simulink model "TST_FlSys_CalcCnvFac"  (R2016b)
settings: Solver=FixedStepDiscrete  StartTime=0.0  StopTime=simTime  FixedStep=sampleTime  RelTol=1e-3
values from neighbouring files (symbols this model uses):
  testCase = 1    [initTST_FlSys_CalcCnvFac_001.m]
libraries: simulink x2
settings Model: Creator=WF305  LastModifiedBy=WF305
settings DebuggingCC: SignalRangeChecking=error

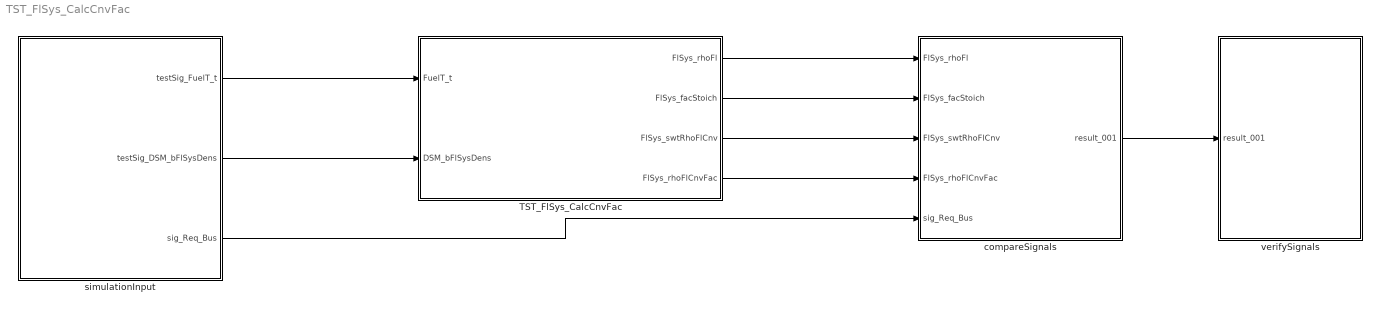
== system TST_FlSys_CalcCnvFac ==
  TST_FlSys_CalcCnvFac : Subsystem
  compareSignals : Subsystem
  simulationInput : Subsystem
  verifySignals : Subsystem
  wires:
  simulationInput/1(testSig_FuelT_t) -> TST_FlSys_CalcCnvFac/1(FuelT_t)
  simulationInput/2(testSig_DSM_bFlSysDens) -> TST_FlSys_CalcCnvFac/2(DSM_bFlSysDens)
  TST_FlSys_CalcCnvFac/1(FlSys_rhoFl) -> compareSignals/1(FlSys_rhoFl)
  TST_FlSys_CalcCnvFac/2(FlSys_facStoich) -> compareSignals/2(FlSys_facStoich)
  TST_FlSys_CalcCnvFac/3(FlSys_swtRhoFlCnv) -> compareSignals/3(FlSys_swtRhoFlCnv)
  TST_FlSys_CalcCnvFac/4(FlSys_rhoFlCnvFac) -> compareSignals/4(FlSys_rhoFlCnvFac)
  simulationInput/3(sig_Req_Bus) -> compareSignals/5(sig_Req_Bus)
  compareSignals/1(result_001) -> verifySignals/1(result_001)

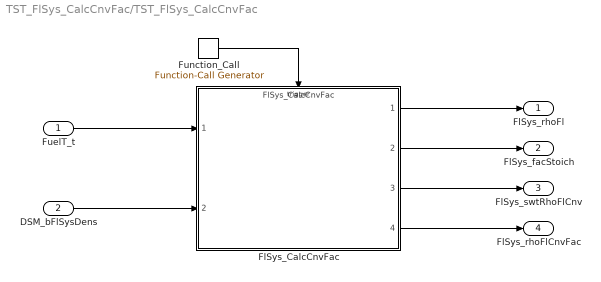
== system TST_FlSys_CalcCnvFac/TST_FlSys_CalcCnvFac ==
  FuelT_t : Inport
  DSM_bFlSysDens : Inport  Port=2
  FlSys_CalcCnvFac : ModelReference  ModelNameDialog=FlSys_CalcCnvFac  ModelReferenceVersion=1.9  TriggerPortName=function  TriggerPortTriggerType=function-call  TriggerPortStatesWhenEnabling=held
  Function_Call : simulink/Ports & Subsystems/Function-Call Generator  sample_time=sampleTime  numberOfIterations=1
  FlSys_rhoFl : Outport
  FlSys_facStoich : Outport  Port=2
  FlSys_swtRhoFlCnv : Outport  Port=3
  FlSys_rhoFlCnvFac : Outport  Port=4
  wires:
  Function_Call/1 -> FlSys_CalcCnvFac/Trigger
  FuelT_t/1 -> FlSys_CalcCnvFac/1
  DSM_bFlSysDens/1 -> FlSys_CalcCnvFac/2
  FlSys_CalcCnvFac/1 -> FlSys_rhoFl/1
  FlSys_CalcCnvFac/2 -> FlSys_facStoich/1
  FlSys_CalcCnvFac/3 -> FlSys_swtRhoFlCnv/1
  FlSys_CalcCnvFac/4 -> FlSys_rhoFlCnvFac/1

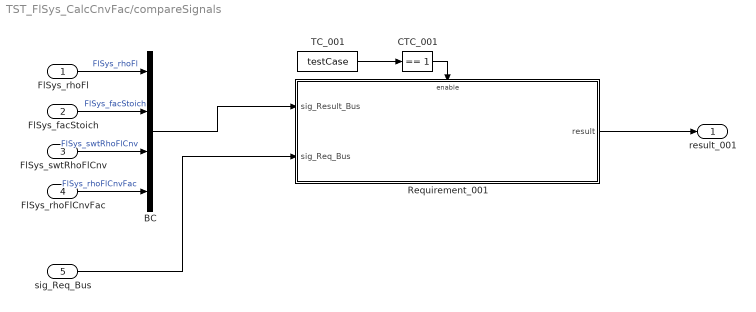
== system TST_FlSys_CalcCnvFac/compareSignals ==
  FlSys_rhoFl : Inport
  FlSys_facStoich : Inport  Port=2
  FlSys_swtRhoFlCnv : Inport  Port=3
  FlSys_rhoFlCnvFac : Inport  Port=4
  sig_Req_Bus : Inport  Port=5
  BC : BusCreator  Inputs=4
  CTC_001 : simulink/Logic and Bit Operations/Compare To Constant  relop===  const=1  OutDataTypeStr=boolean
  Requirement_001 : Subsystem
  TC_001 : Constant  Value=testCase
  result_001 : Outport
  wires:
  FlSys_rhoFl/1 -> BC/1  "FlSys_rhoFl"
  FlSys_facStoich/1 -> BC/2  "FlSys_facStoich"
  FlSys_swtRhoFlCnv/1 -> BC/3  "FlSys_swtRhoFlCnv"
  FlSys_rhoFlCnvFac/1 -> BC/4  "FlSys_rhoFlCnvFac"
  TC_001/1 -> CTC_001/1
  CTC_001/1 -> Requirement_001/Enable
  sig_Req_Bus/1 -> Requirement_001/2(sig_Req_Bus)
  BC/1 -> Requirement_001/1(sig_Result_Bus)
  Requirement_001/1(result) -> result_001/1

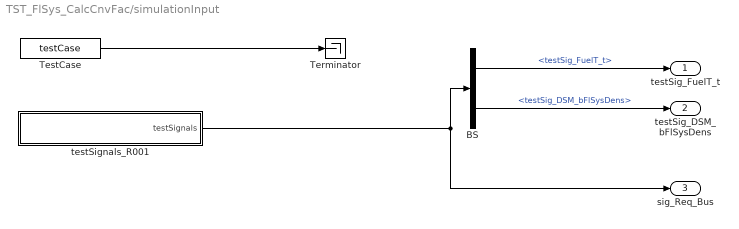
== system TST_FlSys_CalcCnvFac/simulationInput ==
  BS : BusSelector  OutputSignals=testSig_FuelT_t,testSig_DSM_bFlSysDens
  Terminator : Terminator
  TestCase : Constant  Value=testCase
  testSignals_R001 : Subsystem
  testSig_FuelT_t : Outport
  testSig_DSM_bFlSysDens : Outport  Port=2
  sig_Req_Bus : Outport  Port=3
  wires:
  BS/1 -> testSig_FuelT_t/1  "<testSig_FuelT_t>"
  BS/2 -> testSig_DSM_bFlSysDens/1  "<testSig_DSM_bFlSysDens>"
  testSignals_R001/1(testSignals) -> BS/1, sig_Req_Bus/1
  TestCase/1 -> Terminator/1

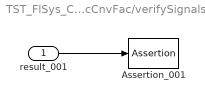
== system TST_FlSys_CalcCnvFac/verifySignals ==
  result_001 : Inport
  Assertion_001 : Assertion
  wires:
  result_001/1 -> Assertion_001/1

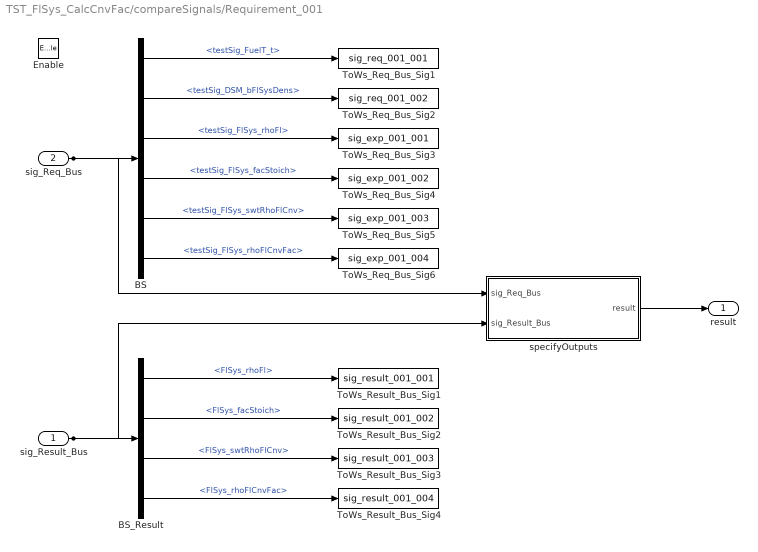
== system TST_FlSys_CalcCnvFac/compareSignals/Requirement_001 ==
  sig_Result_Bus : Inport
  sig_Req_Bus : Inport  Port=2
  Enable : EnablePort
  BS : BusSelector  OutputSignals=testSig_FuelT_t,testSig_DSM_bFlSysDens,testSig_FlSys_rhoFl,testSig_FlSys_facStoich,testSig_FlSys_swtRhoFlCnv,testSig_FlSys_rhoFlCnvFac
  BS_Result : BusSelector  OutputSignals=FlSys_rhoFl,FlSys_facStoich,FlSys_swtRhoFlCnv,FlSys_rhoFlCnvFac
  ToWs_Req_Bus_Sig1 : ToWorkspace  VariableName=sig_req_001_001  SaveFormat=Structure With Time
  ToWs_Req_Bus_Sig2 : ToWorkspace  VariableName=sig_req_001_002  SaveFormat=Structure With Time
  ToWs_Req_Bus_Sig3 : ToWorkspace  VariableName=sig_exp_001_001  SaveFormat=Structure With Time
  ToWs_Req_Bus_Sig4 : ToWorkspace  VariableName=sig_exp_001_002  SaveFormat=Structure With Time
  ToWs_Req_Bus_Sig5 : ToWorkspace  VariableName=sig_exp_001_003  SaveFormat=Structure With Time
  ToWs_Req_Bus_Sig6 : ToWorkspace  VariableName=sig_exp_001_004  SaveFormat=Structure With Time
  ToWs_Result_Bus_Sig1 : ToWorkspace  VariableName=sig_result_001_001  SaveFormat=Structure With Time
  ToWs_Result_Bus_Sig2 : ToWorkspace  VariableName=sig_result_001_002  SaveFormat=Structure With Time
  ToWs_Result_Bus_Sig3 : ToWorkspace  VariableName=sig_result_001_003  SaveFormat=Structure With Time
  ToWs_Result_Bus_Sig4 : ToWorkspace  VariableName=sig_result_001_004  SaveFormat=Structure With Time
  specifyOutputs : Subsystem
  result : Outport
  wires:
  sig_Req_Bus/1 -> BS/1, specifyOutputs/1(sig_Req_Bus)
  BS/1 -> ToWs_Req_Bus_Sig1/1  "<testSig_FuelT_t>"
  BS/2 -> ToWs_Req_Bus_Sig2/1  "<testSig_DSM_bFlSysDens>"
  BS/3 -> ToWs_Req_Bus_Sig3/1  "<testSig_FlSys_rhoFl>"
  BS/4 -> ToWs_Req_Bus_Sig4/1  "<testSig_FlSys_facStoich>"
  BS/5 -> ToWs_Req_Bus_Sig5/1  "<testSig_FlSys_swtRhoFlCnv>"
  BS/6 -> ToWs_Req_Bus_Sig6/1  "<testSig_FlSys_rhoFlCnvFac>"
  sig_Result_Bus/1 -> BS_Result/1, specifyOutputs/2(sig_Result_Bus)
  BS_Result/1 -> ToWs_Result_Bus_Sig1/1  "<FlSys_rhoFl>"
  BS_Result/2 -> ToWs_Result_Bus_Sig2/1  "<FlSys_facStoich>"
  BS_Result/3 -> ToWs_Result_Bus_Sig3/1  "<FlSys_swtRhoFlCnv>"
  BS_Result/4 -> ToWs_Result_Bus_Sig4/1  "<FlSys_rhoFlCnvFac>"
  specifyOutputs/1(result) -> result/1

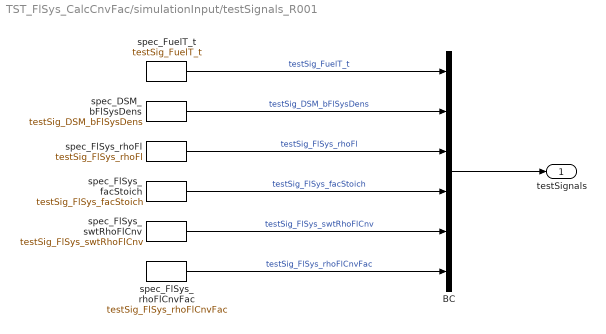
== system TST_FlSys_CalcCnvFac/simulationInput/testSignals_R001 ==
  BC : BusCreator  Inputs=6
  spec_DSM_bFlSysDens : FromWorkspace  VariableName=testSig_DSM_bFlSysDens  Interpolate=off  OutputAfterFinalValue=Holding final value
  spec_FlSys_facStoich : FromWorkspace  VariableName=testSig_FlSys_facStoich  Interpolate=off  OutputAfterFinalValue=Holding final value
  spec_FlSys_rhoFl : FromWorkspace  VariableName=testSig_FlSys_rhoFl  Interpolate=off  OutputAfterFinalValue=Holding final value
  spec_FlSys_rhoFlCnvFac : FromWorkspace  VariableName=testSig_FlSys_rhoFlCnvFac  Interpolate=off  OutputAfterFinalValue=Holding final value
  spec_FlSys_swtRhoFlCnv : FromWorkspace  VariableName=testSig_FlSys_swtRhoFlCnv  Interpolate=off  OutputAfterFinalValue=Holding final value
  spec_FuelT_t : FromWorkspace  VariableName=testSig_FuelT_t  Interpolate=off  OutputAfterFinalValue=Holding final value
  testSignals : Outport
  wires:
  BC/1 -> testSignals/1
  spec_FuelT_t/1 -> BC/1  "testSig_FuelT_t"
  spec_DSM_bFlSysDens/1 -> BC/2  "testSig_DSM_bFlSysDens"
  spec_FlSys_rhoFl/1 -> BC/3  "testSig_FlSys_rhoFl"
  spec_FlSys_facStoich/1 -> BC/4  "testSig_FlSys_facStoich"
  spec_FlSys_swtRhoFlCnv/1 -> BC/5  "testSig_FlSys_swtRhoFlCnv"
  spec_FlSys_rhoFlCnvFac/1 -> BC/6  "testSig_FlSys_rhoFlCnvFac"

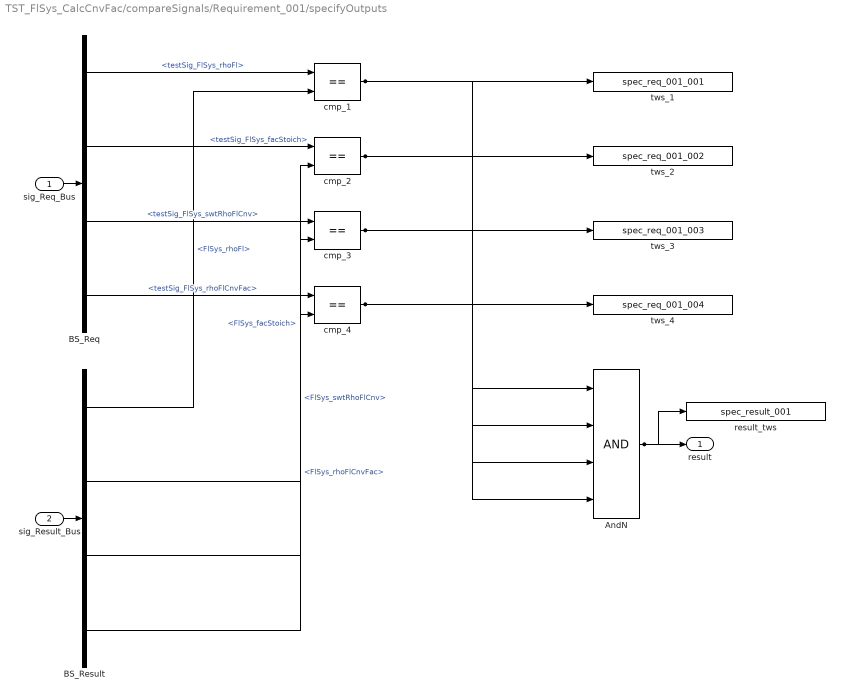
== system TST_FlSys_CalcCnvFac/compareSignals/Requirement_001/specifyOutputs ==
  sig_Req_Bus : Inport
  sig_Result_Bus : Inport  Port=2
  AndN : Logic  Inputs=4
  BS_Req : BusSelector  OutputSignals=testSig_FlSys_rhoFl,testSig_FlSys_facStoich,testSig_FlSys_swtRhoFlCnv,testSig_FlSys_rhoFlCnvFac
  BS_Result : BusSelector  OutputSignals=FlSys_rhoFl,FlSys_facStoich,FlSys_swtRhoFlCnv,FlSys_rhoFlCnvFac
  cmp_{1..4} (4 alike) : RelationalOperator  Operator===  RndMeth=Nearest  InputSameDT=on
  result_tws : ToWorkspace  VariableName=spec_result_001
  tws_1 : ToWorkspace  VariableName=spec_req_001_001
  tws_2 : ToWorkspace  VariableName=spec_req_001_002
  tws_3 : ToWorkspace  VariableName=spec_req_001_003
  tws_4 : ToWorkspace  VariableName=spec_req_001_004
  result : Outport
  wires:
  sig_Req_Bus/1 -> BS_Req/1
  sig_Result_Bus/1 -> BS_Result/1
  AndN/1 -> result/1, result_tws/1
  BS_Req/1 -> cmp_1/1  "<testSig_FlSys_rhoFl>"
  BS_Result/1 -> cmp_1/2  "<FlSys_rhoFl>"
  cmp_1/1 -> tws_1/1, AndN/1
  BS_Req/2 -> cmp_2/1  "<testSig_FlSys_facStoich>"
  BS_Result/2 -> cmp_2/2  "<FlSys_facStoich>"
  cmp_2/1 -> tws_2/1, AndN/2
  BS_Req/3 -> cmp_3/1  "<testSig_FlSys_swtRhoFlCnv>"
  BS_Result/3 -> cmp_3/2  "<FlSys_swtRhoFlCnv>"
  cmp_3/1 -> tws_3/1, AndN/3
  BS_Req/4 -> cmp_4/1  "<testSig_FlSys_rhoFlCnvFac>"
  BS_Result/4 -> cmp_4/2  "<FlSys_rhoFlCnvFac>"
  cmp_4/1 -> tws_4/1, AndN/4
